simulink model "Planta_termica"  (R2022b)
settings: Solver=VariableStepAuto  StartTime=0.0  StopTime=1400  RelTol=1e-3
model workspace (MAT data in the model file):
  rR = 1
undefined symbols (not defined in the file or in its folder): C, R
settings Model: Creator=tengenuzui  LastModifiedBy=tengenuzui

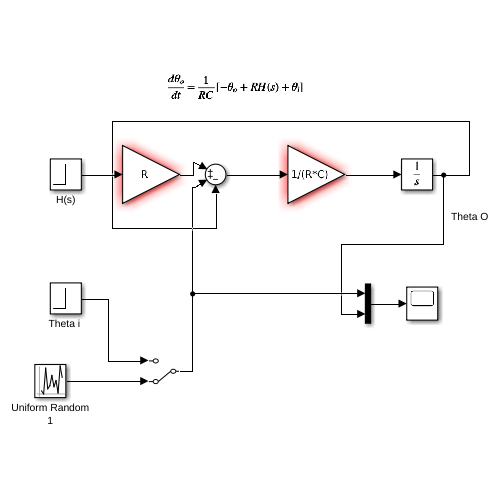
[thumbnail: Simulink's stored preview of the top-level diagram]
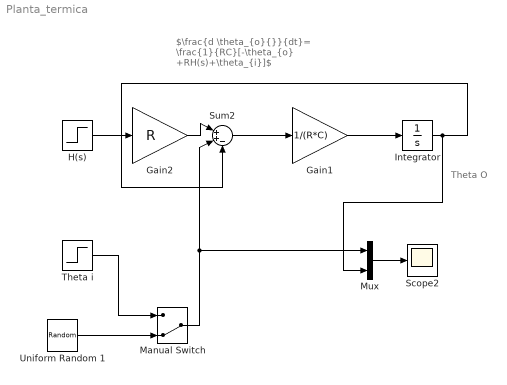
== system Planta_termica ==
  note: $\frac{d \theta_{o}{}}{dt}= \frac{1}{RC}[-\theta_{o} +RH(s)+\theta_{i}]$
  note: Theta O
  Gain1 : Gain  Gain=1/(R*C)
  Gain2 : Gain  Gain=R
  H(s) : Step  Time=10  After=0  SampleTime=0
  Integrator : Integrator
  Manual Switch : ManualSwitch  CurrentSetting=0
  Mux : Mux  Inputs=2
  Scope2 : Scope
  Sum2 : Sum  Inputs=|++-
  "Theta i " : Step  Time=0  Before=25  After=100  SampleTime=140
  Uniform Random 1 : UniformRandomNumber  Minimum=25  Maximum=100  SampleTime=140
  wires:
  Sum2/1 -> Gain1/1
  Gain1/1 -> Integrator/1
  Integrator/1 -> Mux/2, Sum2/3
  Gain2/1 -> Sum2/1
  "Theta i "/1 -> Manual Switch/1
  H(s)/1 -> Gain2/1
  Uniform Random 1/1 -> Manual Switch/2
  Manual Switch/1 -> Sum2/2, Mux/1
  Mux/1 -> Scope2/1
